simulink model "UserSteer_RTW"  (Simulink 9.3)
settings: Solver=ode1  StartTime=0.0  StopTime=inf  FixedStep=0.001  RelTol=1e-3
PreLoadFcn:
  | vehicle = 'Car'; if ~length(which('cmcmd')), cmenv; end
  | UserSteer_RTW_bus
InitFcn:
  | vehicle = 'Car'; if ~length(which('cmcmd')), cmenv; end
  | UserSteer_RTW_bus
libraries: CarMaker4SL x2
Description:
  | CarMaker Plug-in Model Target
settings Model: Creator=IPG  LastModifiedBy=IPG
settings DataIOCC: LimitDataPoints=on
settings OptimizationCC: ExpressionDepthLimit=2147483647
settings DebuggingCC: StateNameClashWarn=warning  SFExecutionAtInitializationDiag=warning
settings HardwareCC: TargetHWDeviceType=32-bit Generic  ProdEqTarget=off
settings RTWCC: SystemTargetFile=CarMaker.tlc  TemplateMakefile=CarMaker_unix-win64.tmf  Description=CarMaker Plug-in Model Target
settings CodeAppCC: MaxIdLength=127
settings STFCustomTargetCC: ModelReferenceCompliant=off  GeneratePreprocessorConditionals=Disable all  MultiInstanceERTCode=on  CodeInterfacePackaging=Reusable function  CPPClassGenCompliant=on  GRTInterface=off  GenerateAllocFcn=on  SystemTargetFile=CarMaker.tlc
settings GRTTargetCC: ModelReferenceCompliant=off  ParMdlRefBuildCompliant=off  CompOptLevelCompliant=off  ConcurrentExecutionCompliant=off  GeneratePreprocessorConditionals=Disable all  MatFileLogging=off  MultiInstanceERTCode=on  CodeInterfacePackaging=Reusable function  GRTInterface=off  GenerateAllocFcn=on  UseToolchainInfoCompliant=off
settings CustomProperty: DataType=string
settings EnumStrPairs: String=Car

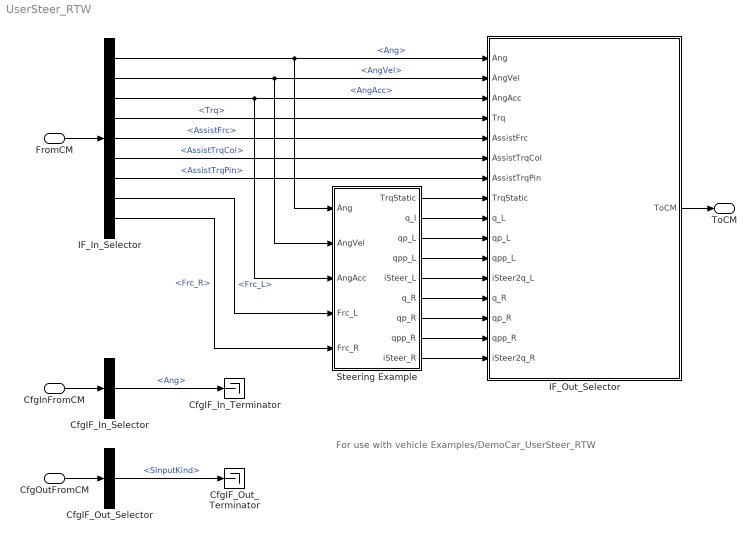
== system UserSteer_RTW ==
  note: For use with vehicle Examples/DemoCar_UserSteer_RTW
  FromCM : Inport  OutDataTypeStr=Bus: cmSteeringIn
  CfgInFromCM : Inport  Port=2  OutDataTypeStr=Bus: cmSteeringCfgIn
  CfgOutFromCM : Inport  Port=3  OutDataTypeStr=Bus: cmSteeringCfgOut
  CfgIF_In_Selector : BusSelector  OutputSignals=Ang
  CfgIF_In_Terminator : Terminator
  CfgIF_Out_Selector : BusSelector  OutputSignals=SInputKind
  CfgIF_Out_Terminator : Terminator
  IF_In_Selector : BusSelector  OutputSignals=Ang,AngVel,AngAcc,Trq,AssistFrc,AssistTrqCol,AssistTrqPin,Frc_L,Frc_R
  IF_Out_Selector : Subsystem  mask(Signal Selection){}
      mask help: Signal Selection Block
      settings: OpenFcn=cmSignalSelect('SignalSelection_CB',gcb)
  Steering Example : Subsystem
  ToCM : Outport  OutDataTypeStr=Bus: cmSteeringOut
  wires:
  FromCM/1 -> IF_In_Selector/1
  IF_Out_Selector/1(ToCM) -> ToCM/1
  CfgInFromCM/1 -> CfgIF_In_Selector/1
  CfgIF_In_Selector/1 -> CfgIF_In_Terminator/1  "<Ang>"
  CfgOutFromCM/1 -> CfgIF_Out_Selector/1
  CfgIF_Out_Selector/1 -> CfgIF_Out_Terminator/1  "<SInputKind>"
  Steering Example/9(iSteer_R) -> IF_Out_Selector/16(iSteer2q_R)
  Steering Example/8(qpp_R) -> IF_Out_Selector/15(qpp_R)
  Steering Example/7(qp_R) -> IF_Out_Selector/14(qp_R)
  Steering Example/6(q_R) -> IF_Out_Selector/13(q_R)
  Steering Example/5(iSteer_L) -> IF_Out_Selector/12(iSteer2q_L)
  Steering Example/4(qpp_L) -> IF_Out_Selector/11(qpp_L)
  Steering Example/3(qp_L) -> IF_Out_Selector/10(qp_L)
  Steering Example/2(q_l) -> IF_Out_Selector/9(q_L)
  Steering Example/1(TrqStatic) -> IF_Out_Selector/8(TrqStatic)
  IF_In_Selector/1 -> Steering Example/1(Ang), IF_Out_Selector/1(Ang)  "<Ang>"
  IF_In_Selector/2 -> Steering Example/2(AngVel), IF_Out_Selector/2(AngVel)  "<AngVel>"
  IF_In_Selector/3 -> Steering Example/3(AngAcc), IF_Out_Selector/3(AngAcc)  "<AngAcc>"
  IF_In_Selector/8 -> Steering Example/4(Frc_L)  "<Frc_L>"
  IF_In_Selector/9 -> Steering Example/5(Frc_R)  "<Frc_R>"
  IF_In_Selector/4 -> IF_Out_Selector/4(Trq)  "<Trq>"
  IF_In_Selector/5 -> IF_Out_Selector/5(AssistFrc)  "<AssistFrc>"
  IF_In_Selector/6 -> IF_Out_Selector/6(AssistTrqCol)  "<AssistTrqCol>"
  IF_In_Selector/7 -> IF_Out_Selector/7(AssistTrqPin)  "<AssistTrqPin>"

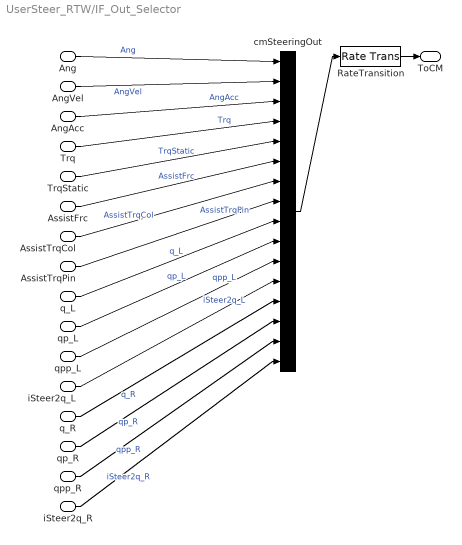
== system UserSteer_RTW/IF_Out_Selector ==
  Ang : Inport
  AngVel : Inport  Port=2
  AngAcc : Inport  Port=3
  Trq : Inport  Port=4
  AssistFrc : Inport  Port=5
  AssistTrqCol : Inport  Port=6
  AssistTrqPin : Inport  Port=7
  TrqStatic : Inport  Port=8
  q_L : Inport  Port=9
  qp_L : Inport  Port=10
  qpp_L : Inport  Port=11
  iSteer2q_L : Inport  Port=12
  q_R : Inport  Port=13
  qp_R : Inport  Port=14
  qpp_R : Inport  Port=15
  iSteer2q_R : Inport  Port=16
  RateTransition : RateTransition  OutPortSampleTime=str2num(get_param(bdroot,'FixedStep'))
  cmSteeringOut : BusCreator  Inputs=16
  ToCM : Outport
  wires:
  RateTransition/1 -> ToCM/1
  cmSteeringOut/1 -> RateTransition/1
  Ang/1 -> cmSteeringOut/1  "Ang"
  AngVel/1 -> cmSteeringOut/2  "AngVel"
  AngAcc/1 -> cmSteeringOut/3  "AngAcc"
  Trq/1 -> cmSteeringOut/4  "Trq"
  AssistFrc/1 -> cmSteeringOut/6  "AssistFrc"
  AssistTrqCol/1 -> cmSteeringOut/7  "AssistTrqCol"
  AssistTrqPin/1 -> cmSteeringOut/8  "AssistTrqPin"
  TrqStatic/1 -> cmSteeringOut/5  "TrqStatic"
  q_L/1 -> cmSteeringOut/9  "q_L"
  qp_L/1 -> cmSteeringOut/10  "qp_L"
  qpp_L/1 -> cmSteeringOut/11  "qpp_L"
  iSteer2q_L/1 -> cmSteeringOut/12  "iSteer2q_L"
  q_R/1 -> cmSteeringOut/13  "q_R"
  qp_R/1 -> cmSteeringOut/14  "qp_R"
  qpp_R/1 -> cmSteeringOut/15  "qpp_R"
  iSteer2q_R/1 -> cmSteeringOut/16  "iSteer2q_R"

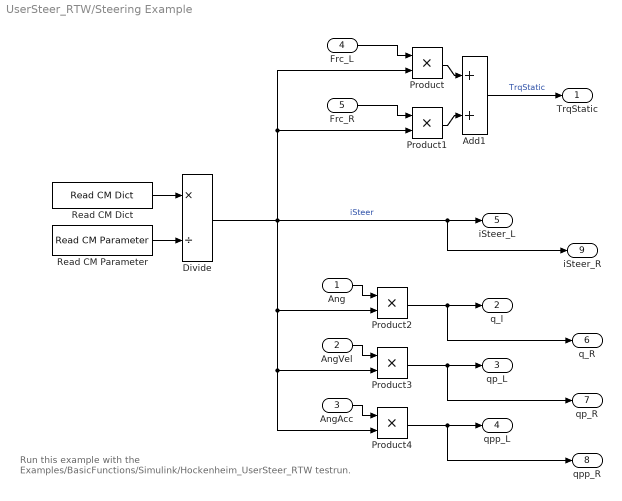
== system UserSteer_RTW/Steering Example ==
  note: Run this example with the
      | Examples/BasicFunctions/Simulink/Hockenheim_UserSteer_RTW testrun.
  Ang : Inport
  AngVel : Inport  Port=2
  AngAcc : Inport  Port=3
  Frc_L : Inport  Port=4
  Frc_R : Inport  Port=5
  Add1 : Sum
  Divide : Product  Inputs=*/
  Product{,1..4} (5 alike) : Product  RndMeth=Zero
  Read CM Dict : CarMaker4SL/Read CM Dict  xname=Steer.Cfg.PosSign  xsync=off
  Read CM Parameter : CarMaker4SL/Read CM Parameter  xfile=Steering  xkey=Steering.Rack2StWhl  xnout=1  xdefaults=[]  xmuxed=on
      settings: SourceProductName=CarMaker4SL
  TrqStatic : Outport
  q_l : Outport  Port=2
  qp_L : Outport  Port=3
  qpp_L : Outport  Port=4
  iSteer_L : Outport  Port=5
  q_R : Outport  Port=6
  qp_R : Outport  Port=7
  qpp_R : Outport  Port=8
  iSteer_R : Outport  Port=9
  wires:
  Product4/1 -> qpp_R/1, qpp_L/1
  AngAcc/1 -> Product4/1
  Product3/1 -> qp_R/1, qp_L/1
  AngVel/1 -> Product3/1
  Product2/1 -> q_R/1, q_l/1
  Ang/1 -> Product2/1
  Divide/1 -> Product1/2, Product/2, iSteer_R/1, iSteer_L/1, Product4/2, Product3/2, Product2/2  "iSteer"
  Frc_R/1 -> Product1/1
  Add1/1 -> TrqStatic/1  "TrqStatic"
  Frc_L/1 -> Product/1
  Product/1 -> Add1/1
  Product1/1 -> Add1/2
  Read CM Dict/1 -> Divide/1
  Read CM Parameter/1 -> Divide/2
